simulink model "a3_4_example_non_linear"  (R2018a)
settings: Solver=VariableStepAuto  StartTime=0.0  StopTime=10.0  RelTol=1e-3
settings Model: Creator=r0x6f736f646f  LastModifiedBy=r0x6f736f646f

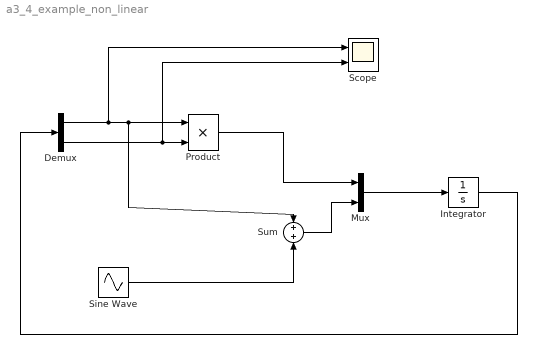
== system a3_4_example_non_linear ==
  Demux : Demux  Outputs=2
  Integrator : Integrator  InitialCondition=[1e05 0.001]
  Mux : Mux  Inputs=2
  Product : Product
  Scope : Scope  NumInputPorts=2
  Sine Wave : Sin  Amplitude=10  SampleTime=0
  Sum : Sum
  wires:
  Mux/1 -> Integrator/1
  Demux/1 -> Product/1, Sum/1, Scope/1
  Demux/2 -> Scope/2, Product/2
  Product/1 -> Mux/1
  Sum/1 -> Mux/2
  Sine Wave/1 -> Sum/2
  Integrator/1 -> Demux/1
